simulink model "proyecto_homeIO"  (R2024b)
settings: Solver=FixedStepAuto  StartTime=0.0  StopTime=450000  FixedStep=200  RelTol=1e-3
values from neighbouring files (symbols this model uses):
  Ad = sysd.A    [mpc.m]
  Ass1 = -4.31323046427e-05    [datos_entrega.mat]    (also in identificacion_ss.m = Sistema.A)
  Ass2 = -4.41902874429e-05    [datos_entrega.mat]    (also in identificacion_ss.m = Sistema3v.A)
  Bd = sysd.B    [mpc.m]
  Bss1 = [1.15391249371e-06 3.71284946538e-07 8.10241189934e-07]    [datos_entrega.mat]    (also in identificacion_ss.m = Sistema.B)
  Bss2 = [-1.29949284091e-06 -4.34702864086e-07]    [datos_entrega.mat]    (also in identificacion_ss.m = Sistema3v.B)
  Cd = sysd.C    [mpc.m]
  Css1 = 89.7044193449    [datos_entrega.mat]    (also in identificacion_ss.m = Sistema.C)
  Css2 = -89.9836686183    [datos_entrega.mat]    (also in identificacion_ss.m = Sistema3v.C)
  Dss1 = [0 0 0]    [datos_entrega.mat]    (also in identificacion_ss.m = Sistema.D)
  Dss2 = [0 0]    [datos_entrega.mat]    (also in identificacion_ss.m = Sistema3v.D)
undefined symbols (not defined in the file or in its folder): D
libraries: mpclib x2, slpidlib x2, realtime_pacer_lib x1
settings Model: Creator=usuario  LastModifiedBy=ferna
settings SolverCC: AlgebraicLoopSolver=TrustRegion
settings DebuggingCC: UnconnectedInputMsg=warning  UnconnectedOutputMsg=warning  UnconnectedLineMsg=warning
settings ModelReferenceCC: EnableRefExpFcnMdlSchedulingChecks=on
settings RTWCC: GPUComputeCapability=3.5  DLArmComputeVersion=19.05

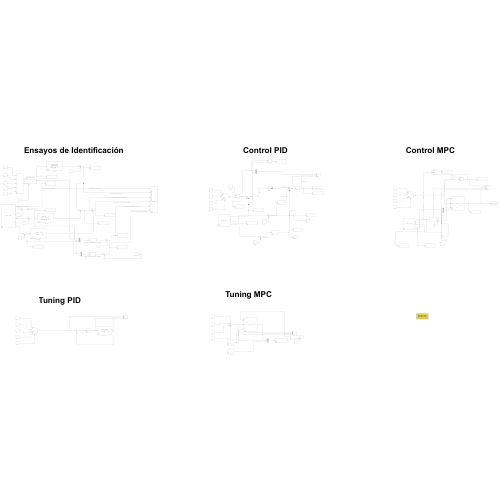
[thumbnail: Simulink's stored preview of the top-level diagram]
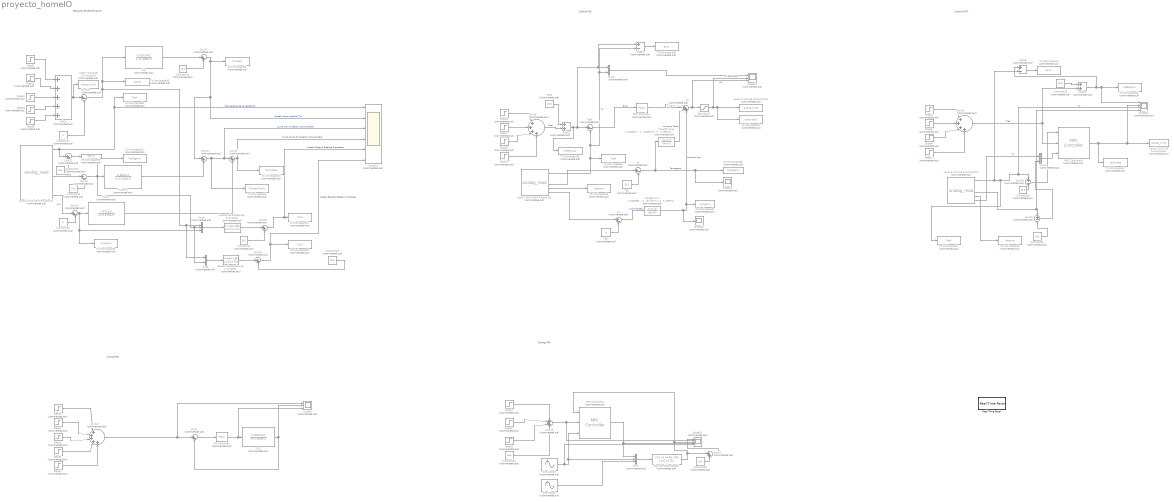
== system proyecto_homeIO ==
  note: Tuning PID
  note: Tuning MPC
  note: Control PID
  note: Ensayos de Identificación
  note: Control MPC
  Add14 : Sum  Commented=on  Inputs=+++++
  Add15 : Sum  Commented=on
  Add16 : Sum  Commented=on  Inputs=+-
  Add17 : Sum  Commented=on
  Add18 : Sum  Commented=on  Inputs=+-
  Constant17 : Constant  Commented=on  Value=0
  Constant{18..19,21..26,28..29} (10 alike) : Constant  Commented=on  Value=16.5
  Constant20 : Constant  Commented=on  Value=0
  Discrete State-Space1 : DiscreteStateSpace  Commented=on  A=Ad  B=Bd  C=Cd  D=D  SampleTime=-1
  Espacio de estadois de 2 variables : StateSpace  Commented=on  A=Ass2  B=Bss2  C=Css2  D=Dss2  InitialCondition=0
  Espacio de estados de 3 variables : StateSpace  Commented=on  A=Ass1  B=Bss1  C=Css1  D=Dss1  InitialCondition=0
  Level-2 MATLAB S-Function11 : M-S-Function  Commented=on  FunctionName=analog_read
  Level-2 MATLAB S-Function14 : M-S-Function  Commented=on  FunctionName=analog_write
  Level-2 MATLAB S-Function15 : M-S-Function  Commented=on  FunctionName=analog_read
  Level-2 MATLAB S-Function16 : M-S-Function  Commented=on  FunctionName=analog_write
  Level-2 MATLAB S-Function18 : M-S-Function  Commented=on  FunctionName=analog_write
  Level-2 MATLAB S-Function19 : M-S-Function  Commented=on  FunctionName=analog_read
  MPC Controller2 : mpclib/MPC Controller  Commented=on  SCDEnableBlockLinearizationSpecification=on  mpcobj=MPCOBJ  is_multiple=0  enable_value=0  return_u0=off  updateMPCinCallerWorkspace=on  md_inport=on  mv_inport=off  uref_inport=off  return_cost=off  return_mvseq=off  return_qpstatus=off  return_xseq=off  return_state=off  return_ovseq=off  state_inport=off  umin_inport=off  umax_inport=off  ymin_inport=off  ymax_inport=off  cc_inport=off  ywt_inport=off  uwt_inport=off  duwt_inport=off  rhoeps_inport=off  pm_inport=off  MaximumP=10  HorizonChoice=FixedHorizon  n_ts=200  n_p=10  n_mv=1  n_md=1  n_ud=0  n_mo=1  n_uo=0  BlockDataType=double  SampleTimeInherited=off  switch_inport=off
  MPC Controller3 : mpclib/MPC Controller  Commented=on  SCDEnableBlockLinearizationSpecification=on  mpcobj=MPCOBJ  is_multiple=0  enable_value=0  return_u0=off  updateMPCinCallerWorkspace=on  md_inport=on  mv_inport=off  uref_inport=off  return_cost=off  return_mvseq=off  return_qpstatus=off  return_xseq=off  return_state=off  return_ovseq=off  state_inport=off  umin_inport=off  umax_inport=off  ymin_inport=off  ymax_inport=off  cc_inport=off  ywt_inport=off  uwt_inport=off  duwt_inport=off  rhoeps_inport=off  pm_inport=off  MaximumP=10  HorizonChoice=FixedHorizon  n_ts=200  n_p=25  n_mv=1  n_md=2  n_ud=0  n_mo=1  n_uo=0  BlockDataType=double  SampleTimeInherited=off  switch_inport=off
  Mux4 : Mux  Commented=on  Inputs=3
  Mux5 : Mux  Commented=on  Inputs=2
  Mux6 : Mux  Commented=on  Inputs=2
  Mux7 : Mux  Commented=on  Inputs=3
  Mux8 : Mux  Commented=on  Inputs=2
  PID Controller : slpidlib/PID Controller  Commented=on  Controller=PID  Form=Parallel  TimeDomain=Continuous-time  UseExternalTs=off  SampleTime=-1  IntegratorMethod=Forward Euler  FilterMethod=Forward Euler  ControllerParametersSource=internal  P=0.503236526924488  I=5.1137309089659e-05  UseKiTs=off  D=-609.888556373582  UseExternalDerivativeSource=off  N=0.000109019708561011  UseFilter=on  TunerSelectOption=Transfer Function Based (PID Tuner App)  InitialConditionSource=internal  InitialConditionForIntegrator=0  InitialConditionForFilter=0  DifferentiatorICPrevScaledInput=0  ExternalReset=none  TrackingMode=off  Kt=1  LimitOutput=off  SatLimitsSource=internal  UpperSaturationLimit=inf  LowerSaturationLimit=-inf  LinearizeAsGain=on  AntiWindupMode=none  Kb=1  LimitIntegrator=off  UpperIntegratorSaturationLimit=inf  LowerIntegratorSaturationLimit=-inf  POutMin=[]  POutMax=[]  IOutMin=[]  IOutMax=[]  DOutMin=[]  DOutMax=[]  NOutMin=[]  NOutMax=[]  SumOutMin=[]  SumOutMax=[]  SaturationOutMin=[]  SaturationOutMax=[]  PParamMin=[]  PParamMax=[]  IParamMin=[]  IParamMax=[]  DParamMin=[]  DParamMax=[]  NParamMin=[]  NParamMax=[]  KbParamMin=[]  KbParamMax=[]  KtParamMin=[]  KtParamMax=[]  KbOutMin=[]  KbOutMax=[]  KtOutMin=[]  KtOutMax=[]  IntegratorOutMin=[]  IntegratorOutMax=[]  FilterOutMin=[]  FilterOutMax=[]  SumI1OutMin=[]  SumI1OutMax=[]  SumI2OutMin=[]  SumI2OutMax=[]  SumI3OutMin=[]  SumI3OutMax=[]  SumI4OutMin=[]  SumI4OutMax=[]  SumDOutMin=[]  SumDOutMax=[]  DifferentiatorOutMin=[]  DifferentiatorOutMax=[]  FilterDiffOutCoefMin=[]  FilterDiffOutCoefMax=[]  ReciprocalOutMin=[]  ReciprocalOutMax=[]  SumDenOutMin=[]  SumDenOutMax=[]  SumNumOutMin=[]  SumNumOutMax=[]  DivideOutMin=[]  DivideOutMax=[]  UdiffTsProdOutMin=[]  UdiffTsProdOutMax=[]  NTsProdOutMin=[]  NTsProdOutMax=[]  UintegralTsProdOutMin=[]  UintegralTsProdOutMax=[]  UngainTsProdOutMin=[]  UngainTsProdOutMax=[]  ClampingZeroOutDataTypeStr=Inherit: Inherit via back propagation  ClampingZeroOutMin=[]  ClampingZeroOutMax=[]  FilterDenConstantOutDataTypeStr=Inherit: Inherit via back propagation  FilterDenConstantOutMin=[]  FilterDenConstantOutMax=[]  PCopyOutDataTypeStr=Inherit: Inherit via back propagation  PCopyOutMin=[]  PCopyOutMax=[]  NCopyOutDataTypeStr=Inherit: Inherit via back propagation  NCopyOutMin=[]  NCopyOutMax=[]  IntegratorContinuousStateAttributes=''  IntegratorStateMustResolveToSignalObject=off  IntegratorRTWStateStorageClass=Auto  FilterContinuousStateAttributes=''  FilterStateMustResolveToSignalObject=off  FilterRTWStateStorageClass=Auto  ParallelPVariant=InternalParameters  IdealPVariant=Disabled  IVariant=InternalParameters  DVariant=InternalParameters  IntegratorVariant=Continuous  SatVariant=Disabled  AWVariant=Passthrough  PCopyVariant=Disabled  TRVariant=Disabled  FdbkBlocksVariant=Forward  IdealPFdbkVariant=Disabled  SatFdbkVariant=Disabled  DerivativeFilterVariant=ContFilter  NVariant=InternalParameters  NCopyVariant=Disabled  FilterICVariant=InternalICsFilter  IntegratorICVariant=InternalICs  ExternalResetVariant=Disabled  TRSumVariant=Passthrough  SumFdbkVariant=Disabled  SumVariant=Sum_PID  TsampFilterVariant=InternalTs  TsampNgainVariant=Passthrough  TsampIntegralVariant=Disabled_SignalSpec  ExternalSaturationOutDataTypeStr=Inherit: Same as second input  DerivativeSourceVariant=ErrorSignal  PreIntVariant=InternalPreInt
  PID Controller4 : slpidlib/PID Controller  Commented=on  Controller=PID  Form=Parallel  TimeDomain=Continuous-time  UseExternalTs=off  SampleTime=-1  IntegratorMethod=Forward Euler  FilterMethod=Forward Euler  ControllerParametersSource=internal  P=4.84895526140258  I=0.00101932449513086  UseKiTs=off  D=-1221.12331406037  UseExternalDerivativeSource=off  N=0.00397089729232935  UseFilter=on  TunerSelectOption=Transfer Function Based (PID Tuner App)  InitialConditionSource=internal  InitialConditionForIntegrator=0  InitialConditionForFilter=0  DifferentiatorICPrevScaledInput=0  ExternalReset=none  TrackingMode=off  Kt=1  LimitOutput=on  SatLimitsSource=internal  UpperSaturationLimit=10  LowerSaturationLimit=0  LinearizeAsGain=on  AntiWindupMode=clamping  Kb=1  LimitIntegrator=off  UpperIntegratorSaturationLimit=inf  LowerIntegratorSaturationLimit=-inf  POutMin=[]  POutMax=[]  IOutMin=[]  IOutMax=[]  DOutMin=[]  DOutMax=[]  NOutMin=[]  NOutMax=[]  SumOutMin=[]  SumOutMax=[]  SaturationOutMin=[]  SaturationOutMax=[]  PParamMin=[]  PParamMax=[]  IParamMin=[]  IParamMax=[]  DParamMin=[]  DParamMax=[]  NParamMin=[]  NParamMax=[]  KbParamMin=[]  KbParamMax=[]  KtParamMin=[]  KtParamMax=[]  KbOutMin=[]  KbOutMax=[]  KtOutMin=[]  KtOutMax=[]  IntegratorOutMin=[]  IntegratorOutMax=[]  FilterOutMin=[]  FilterOutMax=[]  SumI1OutMin=[]  SumI1OutMax=[]  SumI2OutMin=[]  SumI2OutMax=[]  SumI3OutMin=[]  SumI3OutMax=[]  SumI4OutMin=[]  SumI4OutMax=[]  SumDOutMin=[]  SumDOutMax=[]  DifferentiatorOutMin=[]  DifferentiatorOutMax=[]  FilterDiffOutCoefMin=[]  FilterDiffOutCoefMax=[]  ReciprocalOutMin=[]  ReciprocalOutMax=[]  SumDenOutMin=[]  SumDenOutMax=[]  SumNumOutMin=[]  SumNumOutMax=[]  DivideOutMin=[]  DivideOutMax=[]  UdiffTsProdOutMin=[]  UdiffTsProdOutMax=[]  NTsProdOutMin=[]  NTsProdOutMax=[]  UintegralTsProdOutMin=[]  UintegralTsProdOutMax=[]  UngainTsProdOutMin=[]  UngainTsProdOutMax=[]  ClampingZeroOutDataTypeStr=Inherit: Inherit via back propagation  ClampingZeroOutMin=[]  ClampingZeroOutMax=[]  FilterDenConstantOutDataTypeStr=Inherit: Inherit via back propagation  FilterDenConstantOutMin=[]  FilterDenConstantOutMax=[]  PCopyOutDataTypeStr=Inherit: Inherit via back propagation  PCopyOutMin=[]  PCopyOutMax=[]  NCopyOutDataTypeStr=Inherit: Inherit via back propagation  NCopyOutMin=[]  NCopyOutMax=[]  IntegratorContinuousStateAttributes=''  IntegratorStateMustResolveToSignalObject=off  IntegratorRTWStateStorageClass=Auto  FilterContinuousStateAttributes=''  FilterStateMustResolveToSignalObject=off  FilterRTWStateStorageClass=Auto  ParallelPVariant=InternalParameters  IdealPVariant=Disabled  IVariant=InternalParameters  DVariant=InternalParameters  IntegratorVariant=Continuous  SatVariant=Enabled  AWVariant=ContClampingParallel  PCopyVariant=Disabled  TRVariant=Disabled  FdbkBlocksVariant=Forward  IdealPFdbkVariant=Disabled  SatFdbkVariant=Disabled  DerivativeFilterVariant=ContFilter  NVariant=InternalParameters  NCopyVariant=Disabled  FilterICVariant=InternalICsFilter  IntegratorICVariant=InternalICs  ExternalResetVariant=Disabled  TRSumVariant=Passthrough  SumFdbkVariant=Disabled  SumVariant=Sum_PID  TsampFilterVariant=InternalTs  TsampNgainVariant=Passthrough  TsampIntegralVariant=Disabled_SignalSpec  ExternalSaturationOutDataTypeStr=Inherit: Same as second input  DerivativeSourceVariant=ErrorSignal  PreIntVariant=InternalPreInt
  Real-Time Pacer : realtime_pacer_lib/Real-Time Pacer  simTimePerRealTime=5000
      settings: SourceProductName=Real-Time Pacer
  Saturation1 : Saturate  Commented=on  UpperLimit=10  LowerLimit=0
  Scope19 : Scope  Commented=on  NumInputPorts=6
  Scope20 : Scope  Commented=on
  Scope21 : Scope  Commented=on  NumInputPorts=3
  Scope22 : Scope  Commented=on
  Scope23 : Scope  Commented=on  NumInputPorts=5
  Scope24 : Scope  Commented=on  NumInputPorts=4
  Scope8 : Scope  Commented=on  NumInputPorts=3
  Sine Wave1 : Sin  Commented=on  Amplitude=6.5  Bias=16.5  Frequency=72.65e-6  SampleTime=0
  Sine Wave2 : Sin  Commented=on  Amplitude=5  Bias=5  Frequency=72.65e-6  SampleTime=0
  Step10 : Step  Commented=on  Time=0  Before=2  After=0  SampleTime=0
  Step11 : Step  Commented=on  Time=50000  After=3  SampleTime=0
  Step12 : Step  Commented=on  Time=85000  SampleTime=0
  Step13 : Step  Commented=on  Time=190000  Before=2  After=0  SampleTime=0
  Step14 : Step  Commented=on  Time=300000  After=3  SampleTime=0
  Step31 : Step  Commented=on  Time=0  After=0  SampleTime=0
  Step32 : Step  Commented=on  Time=50000  After=2  SampleTime=0
  Step33 : Step  Commented=on  Time=125000  After=2  SampleTime=0
  Step34 : Step  Commented=on  Time=230000  After=2  SampleTime=0
  Step35 : Step  Commented=on  Time=350000  After=3  SampleTime=0
  Step36 : Step  Commented=on  Time=0  Before=0.45  After=0.45  SampleTime=0
  Step37 : Step  Commented=on  Time=75000  After=10  SampleTime=0
  Step38 : Step  Commented=on  Time=200000  After=-7  SampleTime=0
  Step40 : Step  Commented=on  Time=325000  After=5  SampleTime=0
  Step41 : Step  Commented=on  Time=0  After=0  SampleTime=0
  Step42 : Step  Commented=on  Time=160000  After=12  SampleTime=0
  Step43 : Step  Commented=on  Time=300000  After=-6  SampleTime=0
  Step44 : Step  Commented=on  Time=0  Before=0.45  After=0.45  SampleTime=0
  Step45 : Step  Commented=on  Time=75000  After=10  SampleTime=0
  Step46 : Step  Commented=on  Time=200000  After=-7  SampleTime=0
  Step47 : Step  Commented=on  Time=325000  After=5  SampleTime=0
  Sum : Sum  Commented=on  Inputs=|+++++
  Sum{2,16,18..19,22} (5 alike) : Sum  Commented=on  Inputs=|+-
  Sum{17,20..21,23..24,27} (6 alike) : Sum  Commented=on  Inputs=|++
  Sum25 : Sum  Commented=on  Inputs=|++++
  Sum26 : Sum  Commented=on  Inputs=++++
  Sum28 : Sum  Commented=on  Inputs=|++++
  Sum30 : Sum  Commented=on  Inputs=+|-
  Sum31 : Sum  Commented=on  Inputs=+|-
  Teq : Constant  Commented=on  Value=16.5
  Teq2 : Constant  Commented=on  Value=16.5
  Teq7 : Constant  Commented=on  Value=0
  Tl/Lum : TransferFcn  Commented=on  Numerator=[7.471e-5]  Denominator=[1 5.419e-5]
  Tl/Tamb : TransferFcn  Commented=on  Numerator=[3.982e-5]  Denominator=[1 5.185e-5]
  Tl/U : TransferFcn  Commented=on  Numerator=[0.0001402]  Denominator=[1 5.389e-5]
  Tl/U1 : TransferFcn  Commented=on  Numerator=[0.0001402]  Denominator=[1 5.389e-5]
  To Workspace24 : ToWorkspace  Commented=on  VariableName=Tss3  SampleTime=-1
  To Workspace25 : ToWorkspace  Commented=on  VariableName=Tmodelo  SampleTime=-1
  To Workspace26 : ToWorkspace  Commented=on  VariableName=TmodeloTamb  SampleTime=-1
  To Workspace27 : ToWorkspace  Commented=on  VariableName=Tcompleta  SampleTime=-1
  To Workspace28 : ToWorkspace  Commented=on  VariableName=Treal  SampleTime=-1
  To Workspace29 : ToWorkspace  Commented=on  VariableName=Lumgorro  SampleTime=-1
  To Workspace30 : ToWorkspace  Commented=on  VariableName=Ugorro  SampleTime=-1
  To Workspace31 : ToWorkspace  Commented=on  VariableName=Tambgorro  SampleTime=-1
  To Workspace32 : ToWorkspace  Commented=on  VariableName=Tss2  SampleTime=-1
  To Workspace33 : ToWorkspace  Commented=on  VariableName=Tgorro  SampleTime=-1
  To Workspace34 : ToWorkspace  Commented=on  VariableName=Treal  SampleTime=200
  To Workspace35 : ToWorkspace  Commented=on  VariableName=Tambgorro  SampleTime=-1
  To Workspace36 : ToWorkspace  Commented=on  VariableName=Referencia  SampleTime=200
  To Workspace37 : ToWorkspace  Commented=on  VariableName=Usaturada1  SampleTime=200
  To Workspace38 : ToWorkspace  Commented=on  VariableName=Error  SampleTime=200
  To Workspace39 : ToWorkspace  Commented=on  VariableName=Potencia  SampleTime=200
  To Workspace40 : ToWorkspace  Commented=on  VariableName=Lumgorro  SampleTime=-1
  To Workspace41 : ToWorkspace  Commented=on  VariableName=Usaturada  SampleTime=200
  To Workspace42 : ToWorkspace  Commented=on  VariableName=Referencia  SampleTime=200
  To Workspace43 : ToWorkspace  Commented=on  VariableName=Treal  SampleTime=200
  To Workspace44 : ToWorkspace  Commented=on  VariableName=Error  SampleTime=200
  To Workspace46 : ToWorkspace  Commented=on  VariableName=Potencia  SampleTime=200
  Transfer Fcn6 : TransferFcn  Commented=on  Numerator="[-0.284023   -1.5306e-5]"  Denominator="[1   5.185e-5]"
  Transfer Fcn7 : TransferFcn  Commented=on  Numerator="[-0.532882   -2.8717e-5]"  Denominator="[1   5.419e-5]"
  Tref2 : Sum  Commented=on  Inputs=|+-
  s2 : Sum  Commented=on  Inputs=|+++
  s3 : Sum  Commented=on  Inputs=|+-
  s4 : Sum  Commented=on  Inputs=|+-
  wires:
  Constant28/1 -> Sum30/2
  MPC Controller3/1 -> To Workspace41/1, Scope24/2, Level-2 MATLAB S-Function18/1
  Constant29/1 -> Sum31/2
  Sum31/1 -> Mux8/2
  Step46/1 -> Sum28/3
  Step47/1 -> Sum28/4
  Step44/1 -> Sum28/1
  Step45/1 -> Sum28/2
  Sum28/1 -> Add17/2, MPC Controller3/2  "Tref"
  Level-2 MATLAB S-Function19/4 -> Scope24/4, Sum31/1
  Level-2 MATLAB S-Function19/6 -> Mux8/1  "TL"
  Mux8/1 -> MPC Controller3/3
  Constant26/1 -> Add17/1
  Add17/1 -> Add18/1, To Workspace42/1, Scope24/1
  Sum30/1 -> MPC Controller3/1
  Add18/1 -> To Workspace44/1
  Level-2 MATLAB S-Function19/1 -> Add18/2, To Workspace43/1, Scope24/3, Sum30/1  "TL"
  Level-2 MATLAB S-Function19/5 -> To Workspace46/1
  Add15/1 -> To Workspace36/1, Add16/1, Mux6/1, Tref2/1
  s4/1 -> Transfer Fcn7/1  "Luminosidad"
  Step40/1 -> Sum25/4
  Add16/1 -> To Workspace38/1
  Level-2 MATLAB S-Function15/4 -> s3/1
  Step38/1 -> Sum25/3
  Level-2 MATLAB S-Function15/1 -> To Workspace34/1, Add16/2, Mux6/2, Tref2/2  "TL"
  Tref2/1 -> PID Controller4/1  "Error"
  Sum25/1 -> Add15/2  "Tref"
  Teq2/1 -> Add15/1
  Transfer Fcn6/1 -> s2/2  "HL comp Tamb"
  Transfer Fcn7/1 -> Scope22/1, s2/3, To Workspace40/1  "HL comp Lum"
  Teq/1 -> s3/2
  Level-2 MATLAB S-Function15/6 -> s4/1
  Mux6/1 -> Scope21/1
  Teq7/1 -> s4/2
  Saturation1/1 -> Scope21/2, To Workspace37/1, Level-2 MATLAB S-Function16/1  "HL Saturada"
  s3/1 -> Transfer Fcn6/1, Scope20/1, To Workspace35/1  "Tambgorro"
  Level-2 MATLAB S-Function15/5 -> To Workspace39/1
  PID Controller4/1 -> s2/1  "HL Controlador"
  Step37/1 -> Sum25/2
  s2/1 -> Scope21/3, Saturation1/1  "HL"
  Step36/1 -> Sum25/1
  Sum24/1 -> To Workspace32/1, Scope19/6  "Modelo Espacio Estados 2 entradas"
  Step34/1 -> Add14/4
  Level-2 MATLAB S-Function11/4 -> Sum18/1  "Tamb"
  Constant21/1 -> Sum22/2
  Sum17/1 -> Sum20/1, Scope19/2, To Workspace25/1  "Modelo Monovariable Tl/U"
  Constant18/1 -> Sum17/2
  Constant20/1 -> Sum19/2
  Step35/1 -> Add14/5
  Constant23/1 -> Sum24/2
  Espacio de estados de 3 variables/1 -> Sum23/1
  Espacio de estadois de 2 variables/1 -> Sum24/1
  Tl/U/1 -> Sum17/1
  Mux4/1 -> Espacio de estados de 3 variables/1
  Sum23/1 -> To Workspace24/1, Scope19/5  "Modelo Espacio Estados 3 entradas"
  Step32/1 -> Add14/2
  Step33/1 -> Add14/3
  Tl/Lum/1 -> Sum21/2
  Constant17/1 -> Sum16/2
  Level-2 MATLAB S-Function11/1 -> To Workspace28/1, Scope19/1, Sum22/1  "Temperatura de la habitación"
  Tl/Tamb/1 -> Sum20/2
  Sum21/1 -> Scope19/4, To Workspace27/1  "Suma de los 3 modelos monovariable"
  Level-2 MATLAB S-Function11/6 -> Sum19/1  "Lum"
  Constant19/1 -> Sum18/2
  Sum20/1 -> To Workspace26/1, Sum21/1, Scope19/3  "Suma de 2 modelos monovariable"
  Constant22/1 -> Sum23/2
  Sum16/1 -> Mux5/1, Mux4/1, Tl/U/1, To Workspace30/1
  Mux5/1 -> Espacio de estadois de 2 variables/1
  Sum18/1 -> To Workspace31/1, Mux5/2, Mux4/2, Tl/Tamb/1
  Sum22/1 -> To Workspace33/1
  Add14/1 -> Level-2 MATLAB S-Function14/1, Sum16/1
  Sum19/1 -> Mux4/3, To Workspace29/1, Tl/Lum/1
  Step31/1 -> Add14/1
  Tl/U1/1 -> Scope8/2, Sum2/2
  Step13/1 -> Sum/4
  Step10/1 -> Sum/1
  Sum2/1 -> PID Controller/1
  Step14/1 -> Sum/5
  Sum/1 -> Scope8/1, Sum2/1
  PID Controller/1 -> Scope8/3, Tl/U1/1
  Step11/1 -> Sum/2
  Step12/1 -> Sum/3
  MPC Controller2/1 -> Scope23/4, Mux7/1
  Sum26/1 -> Scope23/2, MPC Controller2/2
  Step43/1 -> Sum26/3
  Step41/1 -> Sum26/1
  Step42/1 -> Sum26/2
  Mux7/1 -> Discrete State-Space1/1
  Discrete State-Space1/1 -> Sum27/1, MPC Controller2/1, Scope23/3
  Constant25/1 -> Sum27/2
  Sum27/1 -> Scope23/1
  Sine Wave1/1 -> Scope23/5, MPC Controller2/3, Mux7/2
  Sine Wave2/1 -> Mux7/3
  Constant24/1 -> Sum26/4
